simulink model "Book2221"  (R2019b)
settings: Solver=ode4  StartTime=0.001  StopTime=10.0  FixedStep=0.001  RelTol=1e-3
settings Model: Creator=user  LastModifiedBy=user

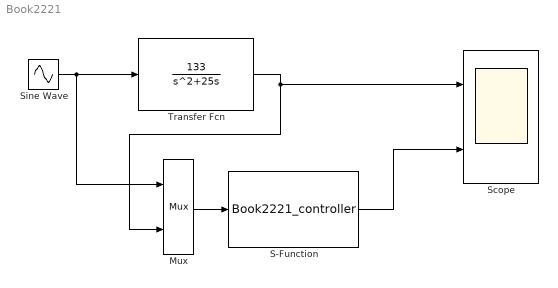
== system Book2221 ==
  Mux : Mux  Inputs=2
  S-Function : S-Function  FunctionName=Book2221_controller  SFunctionDeploymentMode=off  EnableBusSupport=off
  Scope : Scope  NumInputPorts=2
  Sine Wave : Sin  SampleTime=0
  Transfer Fcn : TransferFcn  Numerator=[133]  Denominator=[1 25 0]
  wires:
  Sine Wave/1 -> Mux/1, Transfer Fcn/1
  Transfer Fcn/1 -> Mux/2, Scope/1
  S-Function/1 -> Scope/2
  Mux/1 -> S-Function/1
